simulink model "simpleSwitch"  (Simulink 7.7)
settings: Solver=ode45  StartTime=0.0  StopTime=10.0  RelTol=1e-3
settings Model: Creator=cjz  LastModifiedBy=cjz

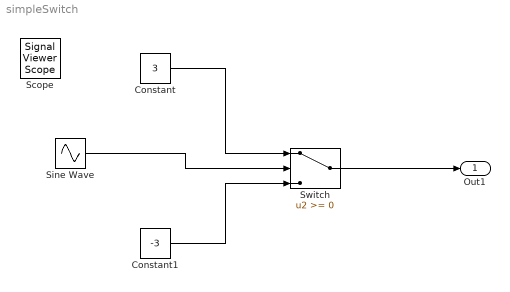
== system simpleSwitch ==
  Constant : Constant  Value=3
  Constant1 : Constant  Value=-3
  Sine Wave : Sin  SampleTime=0
  Switch : Switch
  Out1 : Outport
  Scope : SignalViewerScope  IOType=viewer  NumInputPorts=2  RefreshTime=0.035000
      settings: YMin=-5~-5  YMax=5~5
  wires:
  Constant/1 -> Switch/1
  Sine Wave/1 -> Switch/2
  Constant1/1 -> Switch/3
  Switch/1 -> Out1/1
